simulink model "testando_sensores_hall"  (R2012b)
settings: Solver=ode45  StartTime=0.0  StopTime=3*pi  FixedStep=1e-5  MaxStep=1e-3  RelTol=1e-3
libraries: Encoder x1, BLDC x1
settings Model: Creator=h3now  LastModifiedBy=h3now

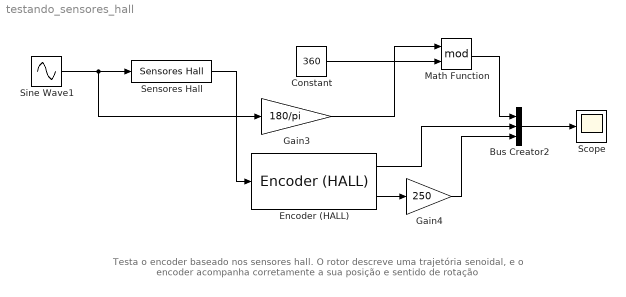
== system testando_sensores_hall ==
  note: Testa o encoder baseado nos sensores hall. O rotor descreve uma trajetória senoidal, e o encoder acompanha
      | corretamente a sua posição e sentido de rotação
  Bus Creator2 : BusCreator  Inputs=3
  Constant : Constant  Value=360
  Encoder (HALL) : Encoder/Encoder (HALL)
  Gain3 : Gain  Gain=180/pi
  Gain4 : Gain  Gain=250
  Math Function : Math  Operator=mod  SaturateOnIntegerOverflow=on
  Scope : Scope
      settings: SaveName=ScopeData7
  Sensores Hall : BLDC/BLDC (block commutation)/Sensores Hall
  Sine Wave1 : Sin  Amplitude=2*pi  SampleTime=0
  wires:
  Sine Wave1/1 -> Gain3/1, Sensores Hall/1
  Sensores Hall/1 -> Encoder (HALL)/1
  Encoder (HALL)/1 -> Bus Creator2/2
  Bus Creator2/1 -> Scope/1
  Gain3/1 -> Math Function/1
  Constant/1 -> Math Function/2
  Math Function/1 -> Bus Creator2/1
  Encoder (HALL)/2 -> Gain4/1
  Gain4/1 -> Bus Creator2/3
